simulink model "egnition_New_updated_shiva"  (R2019b)
settings: Solver=ode1  StartTime=0.0  StopTime=170  FixedStep=0.01  RelTol=1e-3
undefined symbols (not defined in the file or in its folder): BezierCurves, BezierLength, Constants, Driver, Ln, magnitude, v31
libraries: simulink_extras x3, simulink x2
(part 1 of 2)
settings Model: Creator=sivanand.shankar  LastModifiedBy=pradh
settings SolverCC: AlgebraicLoopSolver=LineSearch
settings DataIOCC: ReturnWorkspaceOutputs=off
settings DebuggingCC: ArithmeticOperatorsInVariantConditions=warning
settings SFSimCC: CustomCodeUndefinedFunction=UseInterfaceOnly

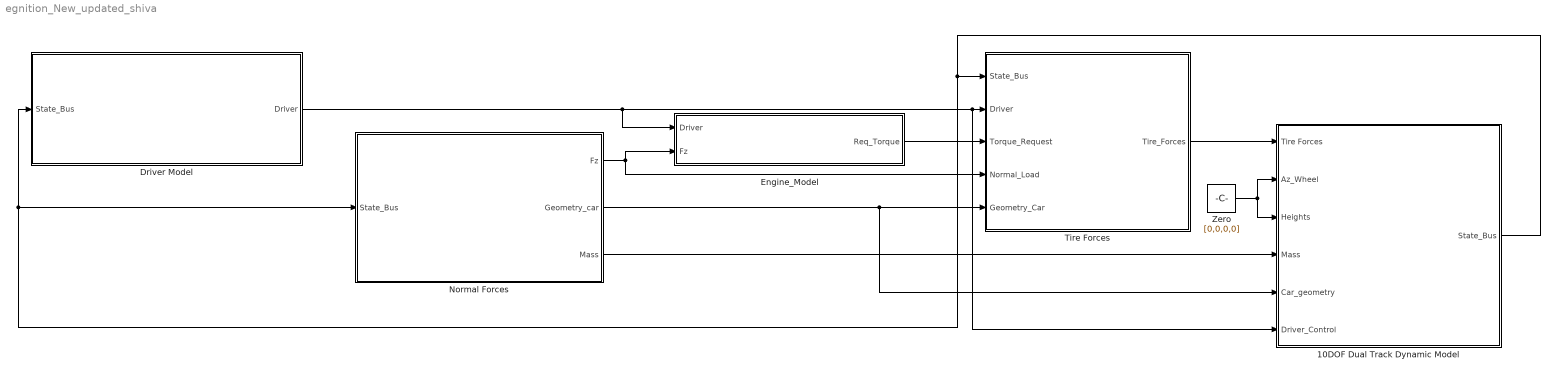
== system egnition_New_updated_shiva ==
  10DOF Dual Track Dynamic Model : Subsystem
  Driver Model : Subsystem
  Engine_Model : Subsystem
  Normal Forces : Subsystem
  "Tire Forces " : Subsystem
  Zero : Constant  Value=[0,0,0,0]
  wires:
  Normal Forces/1(Fz) -> "Tire Forces "/4(Normal_Load), Engine_Model/2(Fz)
  Normal Forces/2(Geometry_car) -> 10DOF Dual Track Dynamic Model/5(Car_geometry), "Tire Forces "/5(Geometry_Car)
  Driver Model/1(Driver) -> Engine_Model/1("Driver "), 10DOF Dual Track Dynamic Model/6(Driver_Control), "Tire Forces "/2(Driver)
  Engine_Model/1(Req_Torque) -> "Tire Forces "/3(Torque_Request)
  "Tire Forces "/1(Tire_Forces) -> 10DOF Dual Track Dynamic Model/1(Tire Forces)
  10DOF Dual Track Dynamic Model/1(State_Bus) -> Driver Model/1(State_Bus), Normal Forces/1(State_Bus), "Tire Forces "/1(State_Bus)
  Zero/1 -> 10DOF Dual Track Dynamic Model/3(Heights), 10DOF Dual Track Dynamic Model/2(Az_Wheel)
  Normal Forces/3(Mass) -> 10DOF Dual Track Dynamic Model/4(Mass)

== system egnition_New_updated_shiva/10DOF Dual Track Dynamic Model ==
  Tire Forces : Inport
  Az_Wheel : Inport  Port=2
  Heights : Inport  Port=3
  Mass : Inport  Port=4
  Car_geometry : Inport  Port=5
  Driver_Control : Inport  Port=6
  Bus Selector : BusSelector  OutputSignals=Fx,Fy
  Vehicle Model : Subsystem
  State_Bus : Outport  VectorParamsAs1DForOutWhenUnconnected=off
  wires:
  Bus Selector/2 -> Vehicle Model/2(Fy)  "<Fy>"
  Bus Selector/1 -> Vehicle Model/1(Fx)  "<Fx>"
  Tire Forces/1 -> Bus Selector/1
  Driver_Control/1 -> Vehicle Model/3(Wheel Angle)
  Heights/1 -> Vehicle Model/7(Heights)
  Mass/1 -> Vehicle Model/6(Mass)
  Az_Wheel/1 -> Vehicle Model/4(Az_Wheel)
  Car_geometry/1 -> Vehicle Model/5(Car_geometry)
  Vehicle Model/1(States Of the Car) -> State_Bus/1

== system egnition_New_updated_shiva/Driver Model ==
  State_Bus : Inport
  Bus Creator : BusCreator  Inputs=3
  Bus Selector : BusSelector  OutputSignals=Velocity.Vx
  Longitudinal Controller : Subsystem  VariantControl=Manual_Driving
  lateral Controller : Subsystem
  Driver : Outport  VectorParamsAs1DForOutWhenUnconnected=off
  wires:
  Longitudinal Controller/2(Brake (0-1)) -> Bus Creator/2  "BrakePos"
  Longitudinal Controller/1(Throttle (0-1)) -> Bus Creator/1  "ThrottlePos"
  State_Bus/1 -> lateral Controller/1("Input Bus "), Bus Selector/1
  Bus Creator/1 -> Driver/1
  Bus Selector/1 -> Longitudinal Controller/1(Drive Velocity)  "<Vx>"
  lateral Controller/1(Steering_Angle) -> Bus Creator/3  "WheelAngle"
  lateral Controller/2(Output) -> Longitudinal Controller/2(length)

== system egnition_New_updated_shiva/Engine_Model ==
  "Driver " : Inport
  Fz : Inport  Port=2
  Add : Sum  Inputs=4
  Bus Creator : BusCreator  Inputs=4
  Bus Selector : BusSelector  OutputSignals=Fz_total.FZ_FL,Fz_total.FZ_FR,Fz_total.FZ_RL,Fz_total.FZ_RR
  Bus Selector1 : BusSelector  OutputSignals=ThrottlePos,BrakePos
  Divide{,1..3} (4 alike) : Product  Inputs=*/
  MATLAB Function : MATLAB Function  TreatAsAtomicUnit=on
  Max Torque for the Car(Nm) : Constant  Value=Constants.driving_param.front_peak_torque*4
  Product{,1..3} (4 alike) : Product
  Saturation{,1..3} (4 alike) : Saturate  UpperLimit=Constants.driving_param.front_peak_torque  LowerLimit=-Constants.driving_param.front_peak_torque
  Scope : Scope  NumInputPorts=4
  Req_Torque : Outport  VectorParamsAs1DForOutWhenUnconnected=off
  wires:
  Saturation1/1 -> Scope/2, Bus Creator/2  "Vectored Torque FR"
  Bus Creator/1 -> Req_Torque/1
  Product1/1 -> Saturation1/1
  Bus Selector/1 -> Divide/1, Add/1  "<FZ_FL>"
  Product2/1 -> Saturation2/1
  Saturation/1 -> Scope/1, Bus Creator/1  "Vectored Torque FL"
  Product3/1 -> Saturation3/1
  Saturation3/1 -> Scope/4, Bus Creator/4  "Vectored Torque RR"
  Product/1 -> Saturation/1
  Divide2/1 -> Product2/1
  Saturation2/1 -> Scope/3, Bus Creator/3  "Vectored Torque RL"
  Bus Selector/2 -> Divide1/1, Add/2  "<FZ_FR>"
  Divide/1 -> Product/1
  Add/1 -> Divide1/2, Divide/2, Divide2/2, Divide3/2
  Bus Selector/4 -> Divide3/1, Add/4  "<FZ_RR>"
  Divide3/1 -> Product3/1
  Divide1/1 -> Product1/1
  Bus Selector/3 -> Divide2/1, Add/3  "<FZ_RL>"
  Fz/1 -> Bus Selector/1
  Max Torque for the Car(Nm)/1 -> MATLAB Function/3(T_peak)
  Bus Selector1/1 -> MATLAB Function/1(TP)  "<ThrottlePos>"
  Bus Selector1/2 -> MATLAB Function/2(BP)  "<BrakePos>"
  "Driver "/1 -> Bus Selector1/1
  MATLAB Function/1(Requested_Torque) -> Product/2, Product1/2, Product3/2, Product2/2

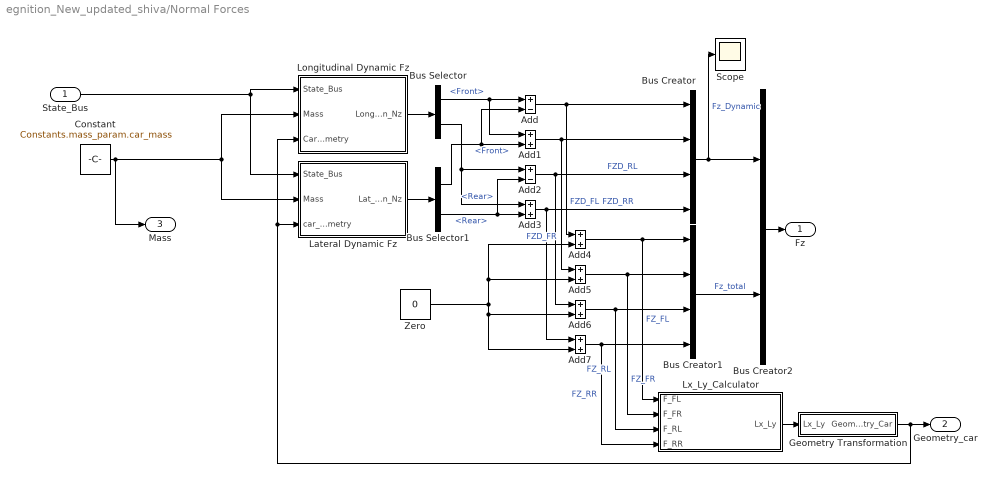
== system egnition_New_updated_shiva/Normal Forces ==
  State_Bus : Inport
  Add : Sum  Inputs=+-
  Add{1,3..7} (6 alike) : Sum
  Add2 : Sum  Inputs=+-
  Bus Creator : BusCreator  Inputs=4
  Bus Creator1 : BusCreator  Inputs=4
  Bus Creator2 : BusCreator  Inputs=2
  Bus Selector : BusSelector  OutputSignals=Front,Rear
  Bus Selector1 : BusSelector  OutputSignals=Front,Rear
  Constant : Constant  Value=Constants.mass_param.car_mass
  Geometry Transformation : Subsystem
  Lateral Dynamic Fz : Subsystem  mask{a_s=Constants.dim_param_mass.distance_of_sprung_cg_from_rear_axle, W_s=Constants.mass_param.sprung_mass, K_F=Constants.roll_param.front_roll_stiffness, L_cgr=Constants.dim_param_mass.distance_sprung_mass_cg_and_roll_axis, K_R=Constants.roll_param.rear_roll_stiffness, H_s=Constants.dim_param_mass.height_front_unsprung_cg, Z_RF=Constants.roll_param.front_roll_center_height, Z_RR=Constants.roll_param.rear_roll_center_height, W_uF=Constants.mass_param.front_unsprung_mass, W_uR=Constants.mass_param.rear_unsprung_mass, Z_uF=Constants.dim_param_mass.height_front_unsprung_cg, Z_uR=Constants.dim_param_mass.height_rear_unsprung_cg}
      mask prompts: a_s "Distance of sprung cg from rear axle"; W_s "Sprung Mass"; K_F "Front Roll Stiffness"; L_cgr "Distance from Sprung mass CG to Roll Axis"; K_R "Rear Roll Stiffness"; H_s "Unsprung Mass CG Height"; Z_RF "Roll Centric Height Front"; Z_RR "Roll Centric Height Rear"; W_uF "Front UnSprung Mass"; W_uR "Rear UnSprung Mass"; Z_uF "Front Unsprung CG Height"; Z_uR "Rear Unsprung CG Height"
  Longitudinal Dynamic Fz : Subsystem  mask{CG_Height=Constants.dim_param.cg_height}
      mask prompts: CG_Height "Height CoG"
  Lx_Ly_Calculator : Subsystem  mask{wb=Constants.dim_param.wheel_base, wt_FA=Constants.dim_param.front_track, wt_RA=Constants.dim_param.rear_track}
      mask prompts: wb "Wheel base [m]"; wt_FA "Wheel track [m] - front axle"; wt_RA "Wheel track [m] - rear axle"
      mask DialogControl DescGroupVar Prompt: Corner position calculation
      mask DialogControl DescTextVar Prompt: Calculates the height of the vehicle corners based on the height, the roll angle and the pitch at the center of gravity
  Scope : Scope
  Zero : Constant  Value=0  OutDataTypeStr=Inherit: Inherit via back propagation
  Fz : Outport  VectorParamsAs1DForOutWhenUnconnected=off
  Geometry_car : Outport  Port=2  VectorParamsAs1DForOutWhenUnconnected=off
  Mass : Outport  Port=3  VectorParamsAs1DForOutWhenUnconnected=off
  wires:
  Geometry Transformation/1(Geometry_Car) -> Geometry_car/1, Lateral Dynamic Fz/3(car_Geometry), Longitudinal Dynamic Fz/3(Car_Geometry)
  Lx_Ly_Calculator/1(Lx_Ly) -> Geometry Transformation/1(Lx_Ly)
  Bus Creator2/1 -> Fz/1
  Bus Creator/1 -> Scope/1, Bus Creator2/1  "Fz_Dynamic"
  Bus Selector1/1 -> Add1/2, Add/2  "<Front>"
  Bus Selector1/2 -> Add3/2, Add2/2  "<Rear>"
  Add1/1 -> Bus Creator/2, Add5/1  "FZD_FR"
  Add2/1 -> Bus Creator/3, Add6/1  "FZD_RL"
  Add3/1 -> Bus Creator/4, Add7/1  "FZD_RR"
  Bus Selector/2 -> Add3/1, Add2/1  "<Rear>"
  Bus Selector/1 -> Add/1, Add1/1  "<Front>"
  Lateral Dynamic Fz/1(Lat_Dyn_Nz) -> Bus Selector1/1
  Longitudinal Dynamic Fz/1(Long_Dyn_Nz) -> Bus Selector/1
  State_Bus/1 -> Lateral Dynamic Fz/1(State_Bus), Longitudinal Dynamic Fz/1(State_Bus)
  Add4/1 -> Bus Creator1/1, Lx_Ly_Calculator/1(F_FL)  "FZ_FL"
  Add5/1 -> Bus Creator1/2, Lx_Ly_Calculator/2(F_FR)  "FZ_FR"
  Add6/1 -> Bus Creator1/3, Lx_Ly_Calculator/3(F_RL)  "FZ_RL"
  Add7/1 -> Bus Creator1/4, Lx_Ly_Calculator/4(F_RR)  "FZ_RR"
  Add/1 -> Add4/1, Bus Creator/1  "FZD_FL"
  Bus Creator1/1 -> Bus Creator2/2  "Fz_total"
  Constant/1 -> Mass/1, Lateral Dynamic Fz/2(Mass), Longitudinal Dynamic Fz/2(Mass)
  Zero/1 -> Add7/2, Add6/2, Add5/2, Add4/2

== system egnition_New_updated_shiva/Tire Forces  ==
  State_Bus : Inport
  Driver : Inport  Port=2
  Torque_Request : Inport  Port=3
  Normal_Load : Inport  Port=4
  Geometry_Car : Inport  Port=5
  Bus Creator : BusCreator  Inputs=2
  Tire Model : Subsystem  mask{Radius=Constants.wheel_param.wheel_radius}
      mask prompts: Radius "Radius of the wheel"
  Tire_Forces : Outport  VectorParamsAs1DForOutWhenUnconnected=off
  wires:
  Tire Model/1(Fx) -> Bus Creator/1  "Fx"
  Bus Creator/1 -> Tire_Forces/1
  Tire Model/2(Fy) -> Bus Creator/2  "Fy"
  Normal_Load/1 -> Tire Model/5(Nz)
  Torque_Request/1 -> Tire Model/4(Req Torrque)
  Driver/1 -> Tire Model/3(Driver)
  Geometry_Car/1 -> Tire Model/2(Geometry_Car)
  State_Bus/1 -> Tire Model/1(State Bus)

== system egnition_New_updated_shiva/10DOF Dual Track Dynamic Model/Vehicle Model ==
  Fx : Inport
  Fy : Inport  Port=2
  Wheel Angle : Inport  Port=3
  Az_Wheel : Inport  Port=4
  Car_geometry : Inport  Port=5
  Mass : Inport  Port=6
  Heights : Inport  Port=7
  Bus Creator : BusCreator  Inputs=2
  Bus Creator1 : BusCreator  Inputs=3
  Bus Creator2 : BusCreator  Inputs=3
  Bus Creator3 : BusCreator  Inputs=3
  Bus Creator4 : BusCreator  Inputs=4
  Bus Creator5 : BusCreator  Inputs=2
  Bus Selector : BusSelector  OutputSignals=WheelAngle
  "Roll And Pitch " : Subsystem  mask{Ts=25}
      mask prompts: Ts "Sampling Time of the car sensors"
  Vehicle Model : Subsystem  mask{Jz=Constants.other_param.Moment_of_Inertia, Radius=Constants.wheel_param.wheel_radius}
      mask prompts: Jz "Moment of Inertia around Z axis"; Radius "Radius of the tire"
      mask TypeOptions Jz: Moment_of_Inertia_Z/Value
  States Of the Car : Outport  VectorParamsAs1DForOutWhenUnconnected=off
  wires:
  Az_Wheel/1 -> Vehicle Model/6(Az)
  Mass/1 -> Vehicle Model/5(Mass)
  Car_geometry/1 -> Vehicle Model/4(Car_Geometry)
  Fy/1 -> Vehicle Model/2("Fy ")
  Fx/1 -> Vehicle Model/1(Fx)
  Vehicle Model/4(Velocity_Y) -> Bus Creator1/2  "Vy"
  Vehicle Model/3(Velocity_X) -> Bus Creator1/1  "Vx"
  Vehicle Model/5(Yaw Rate) -> Bus Creator1/3  "Psi_Dot"
  Vehicle Model/1(Acceleration_X) -> Bus Creator/1  "Ax"
  Bus Creator/1 -> Bus Creator4/1  "Acceleration"
  Bus Creator1/1 -> Bus Creator4/2  "Velocity"
  Bus Creator2/1 -> Bus Creator4/3  "Position"
  Bus Creator4/1 -> States Of the Car/1
  Wheel Angle/1 -> Bus Selector/1
  Bus Selector/1 -> Vehicle Model/3(Wheel_Angle)  "<WheelAngle>"
  Vehicle Model/7(Position_Y) -> Bus Creator2/2  "Y"
  Vehicle Model/6(Position_X) -> Bus Creator2/1  "X"
  Vehicle Model/8(Position_Z) -> Bus Creator2/3  "Z"
  Vehicle Model/9(Yaw Angle) -> Bus Creator3/1  "Psi"
  Heights/1 -> "Roll And Pitch "/1(Heights)
  Vehicle Model/2(Acceleration_Y) -> Bus Creator/2  "Ay"
  Bus Creator3/1 -> Bus Creator4/4  "Angle"
  Bus Creator5/1 -> Vehicle Model/7(Roll and Pitch)  "Angle"
  "Roll And Pitch "/1(Pitch) -> Bus Creator5/1, Bus Creator3/2  "Theta"
  "Roll And Pitch "/2(Roll) -> Bus Creator5/2, Bus Creator3/3  "Phi"

== system egnition_New_updated_shiva/Driver Model/Longitudinal Controller ==
  note: Velocity Input
  Drive Velocity : Inport
  length : Inport  Port=2
  1-D Lookup Table : Lookup_n-D  NumberOfTableDimensions=1  BreakpointsForDimension1=Ln  Table=v31  InternalRulePriority=Speed  RndMeth=Simplest  InputSameDT=on
  B % to Decimal : Gain  Gain=-0.01
  Brake extractor : Saturate  UpperLimit=0  LowerLimit=-100
  Constant1 : Constant  Value=1.53
  Initialization : Step  Time=Constants.initial_param.initialization_velocity  After=Constants.initial_param.step_val
  Longitudinal PID : simulink/Continuous/PID Controller  Controller=PI  Form=Parallel  TimeDomain=Continuous-time  SampleTime=-1  IntegratorMethod=Forward Euler  FilterMethod=Forward Euler  ControllerParametersSource=internal  P=50  I=2  D=Driver.Long.PID.Kd  UseFilter=on  N=Driver.Long.PID.N  TunerSelectOption=Transfer Function Based (PID Tuner App)  InitialConditionSource=internal  InitialConditionForIntegrator=0  InitialConditionForFilter=0  DifferentiatorICPrevScaledInput=0  ExternalReset=none  TrackingMode=off  Kt=1  LimitOutput=off  UpperSaturationLimit=inf  LowerSaturationLimit=-inf  LinearizeAsGain=on  AntiWindupMode=none  Kb=1  POutMin=[]  POutMax=[]  IOutMin=[]  IOutMax=[]  DOutMin=[]  DOutMax=[]  NOutMin=[]  NOutMax=[]  SumOutMin=[]  SumOutMax=[]  SaturationOutMin=[]  SaturationOutMax=[]  PParamMin=[]  PParamMax=[]  IParamMin=[]  IParamMax=[]  DParamMin=[]  DParamMax=[]  NParamMin=[]  NParamMax=[]  KbParamMin=[]  KbParamMax=[]  KtParamMin=[]  KtParamMax=[]  KbOutMin=[]  KbOutMax=[]  KtOutMin=[]  KtOutMax=[]  IntegratorOutMin=[]  IntegratorOutMax=[]  FilterOutMin=[]  FilterOutMax=[]  SumI1OutMin=[]  SumI1OutMax=[]  SumI2OutMin=[]  SumI2OutMax=[]  SumI3OutMin=[]  SumI3OutMax=[]  SumI4OutMin=[]  SumI4OutMax=[]  SumDOutMin=[]  SumDOutMax=[]  DifferentiatorOutMin=[]  DifferentiatorOutMax=[]  FilterDiffOutCoefMin=[]  FilterDiffOutCoefMax=[]  ReciprocalOutMin=[]  ReciprocalOutMax=[]  SumDenOutMin=[]  SumDenOutMax=[]  SumNumOutMin=[]  SumNumOutMax=[]  DivideOutMin=[]  DivideOutMax=[]  IntegratorContinuousStateAttributes=''  IntegratorStateMustResolveToSignalObject=off  IntegratorRTWStateStorageClass=Auto  FilterContinuousStateAttributes=''  FilterStateMustResolveToSignalObject=off  FilterRTWStateStorageClass=Auto  ParallelPVariant=InternalParameters  IdealPVariant=Disabled  IVariant=InternalParameters  DVariant=Disabled  IntegratorVariant=Continuous  SatVariant=Disabled  AWVariant=Passthrough  PCopyVariant=Disabled  TRVariant=Disabled  FdbkBlocksVariant=Forward  IdealPFdbkVariant=Disabled  SatFdbkVariant=Disabled  DerivativeFilterVariant=Disabled  NVariant=Disabled  NCopyVariant=Disabled_SignalSpec  FilterICVariant=Disabled  IntegratorICVariant=InternalICs  ExternalResetVariant=Disabled  TRSumVariant=Passthrough  SumFdbkVariant=Disabled  SumVariant=Sum_PI
  Manual Input : Constant  Value=35
  Manual Switch : ManualSwitch  CurrentSetting=0
  Max_Velocity Saturation : Saturate  UpperLimit=50  LowerLimit=0
  Product : Product
  Scope1 : Scope
  Scope2 : Scope
  Sum : Sum  Inputs=-+
  Sum1 : Sum  Inputs=|++
  T % to Decimal : Gain  Gain=0.01
  Throttle extractor : Saturate  UpperLimit=100  LowerLimit=0
  kmph to mps : Gain  Gain=1/3.6
  kmph to mps2 : Gain  Gain=3.6
  Throttle (0-1) : Outport  VectorParamsAs1DForOutWhenUnconnected=off
  Brake (0-1) : Outport  Port=2  VectorParamsAs1DForOutWhenUnconnected=off
  wires:
  Product/1 -> Max_Velocity Saturation/1, Scope1/1
  Throttle extractor/1 -> T % to Decimal/1
  Longitudinal PID/1 -> Brake extractor/1, Throttle extractor/1
  Brake extractor/1 -> B % to Decimal/1
  kmph to mps/1 -> Product/1  "Reference Speed"
  Manual Switch/1 -> kmph to mps/1
  Manual Input/1 -> Manual Switch/2
  Initialization/1 -> Product/2
  B % to Decimal/1 -> Brake (0-1)/1
  Max_Velocity Saturation/1 -> Sum/2
  Sum/1 -> Longitudinal PID/1
  Drive Velocity/1 -> Sum/1  "Actual_Speed"
  T % to Decimal/1 -> Scope2/1, Throttle (0-1)/1
  1-D Lookup Table/1 -> kmph to mps2/1  "Reference Speed"
  Sum1/1 -> 1-D Lookup Table/1
  Constant1/1 -> Sum1/2
  length/1 -> Sum1/1
  kmph to mps2/1 -> Manual Switch/1  "Reference Speed"

== system egnition_New_updated_shiva/Driver Model/lateral Controller ==
  "Input Bus " : Inport
  BezierPathReference : MATLAB Function  TreatAsAtomicUnit=on
  Bus Selector : BusSelector  OutputSignals=Angle.Psi
  Bus Selector1 : BusSelector  OutputSignals=Position.X,Position.Y,Position.Z
  Bus Selector2 : BusSelector  OutputSignals=Velocity.Psi_Dot
  Bus Selector3 : BusSelector  OutputSignals=Velocity.Vx
  Bus Selector4 : BusSelector  OutputSignals=Angle.Psi
  Constant : Constant  Value=0.001
  Constant1 : Constant  Value=BezierCurves
  Constant2 : Constant  Value=BezierLength
  IC{,1..2,4} (4 alike) : InitialCondition  Value=0
  IC3 : InitialCondition  Value=[0;0;0]
  Mux : Mux  Inputs=3
  Scope2 : Scope  NumInputPorts=3
  Subsystem : Subsystem
  Steering_Angle : Outport  VectorParamsAs1DForOutWhenUnconnected=off
  Output : Outport  Port=2
  wires:
  BezierPathReference/1(ey) -> IC/1, Scope2/1  "ey"
  Constant1/1 -> BezierPathReference/4(bezierCurves)
  IC3/1 -> BezierPathReference/1(pCar)
  "Input Bus "/1 -> Bus Selector3/1, Bus Selector4/1, Bus Selector2/1, Bus Selector1/1, Bus Selector/1
  Mux/1 -> IC3/1
  IC1/1 -> Subsystem/2(e_gamma)
  IC2/1 -> BezierPathReference/2(yawCar)
  Bus Selector1/3 -> Mux/3  "<Z>"
  Bus Selector/1 -> IC2/1  "<Psi>"
  BezierPathReference/2(eYaw) -> IC1/1, Scope2/2  "eyaw"
  IC/1 -> Subsystem/1(ey)
  Constant2/1 -> BezierPathReference/5(bezierLength)
  Bus Selector1/1 -> Mux/1  "<X>"
  Constant/1 -> BezierPathReference/3(tol)
  Bus Selector1/2 -> Mux/2  "<Y>"
  BezierPathReference/3(kappa) -> IC4/1, Scope2/3
  IC4/1 -> Subsystem/3(kappa)
  Bus Selector2/1 -> Subsystem/4(psi_dot)  "<Psi_Dot>"
  Bus Selector3/1 -> Subsystem/5(dx_C_dt)  "<Vx>"
  Bus Selector4/1 -> Subsystem/6(psi)  "<Psi>"
  Subsystem/1(delta_fb) -> Steering_Angle/1
  BezierPathReference/4(lengh) -> Output/1  "length"

== system egnition_New_updated_shiva/Normal Forces/Geometry Transformation ==
  Lx_Ly : Inport
  Bus Creator : BusCreator  Inputs=5
  Constant : Constant  Value=Constants.dim_param.dist_cg_front
  Constant1 : Constant  Value=Constants.dim_param.dist_cg_rear
  Constant2 : Constant  Value=Constants.dim_param.front_track
  Constant3 : Constant  Value=Constants.dim_param.rear_track
  Constant4 : Constant  Value=Constants.dim_param.wheel_base
  Terminator : Terminator
  Geometry_Car : Outport  VectorParamsAs1DForOutWhenUnconnected=off
  wires:
  Bus Creator/1 -> Geometry_Car/1
  Constant/1 -> Bus Creator/1  "Lf"
  Constant1/1 -> Bus Creator/2  "Lr"
  Constant2/1 -> Bus Creator/3  "Tf"
  Constant3/1 -> Bus Creator/4  "Tr"
  Constant4/1 -> Bus Creator/5  "Wb"
  Lx_Ly/1 -> Terminator/1

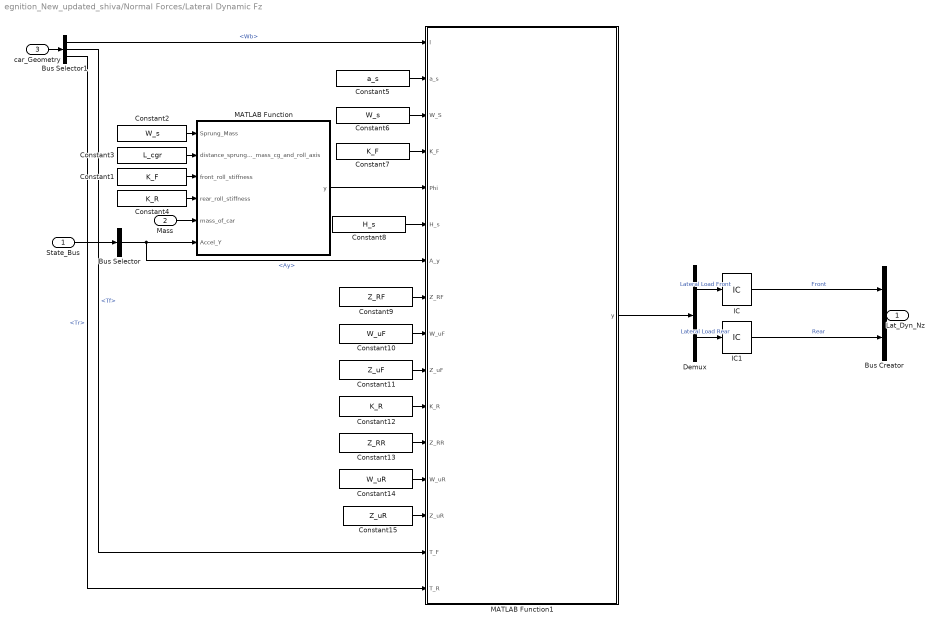
== system egnition_New_updated_shiva/Normal Forces/Lateral Dynamic Fz ==
  State_Bus : Inport
  Mass : Inport  Port=2
  car_Geometry : Inport  Port=3
  Bus Creator : BusCreator  Inputs=2
  Bus Selector : BusSelector  OutputSignals=Acceleration.Ay
  Bus Selector1 : BusSelector  OutputSignals=Wb,Tf,Tr
  Constant1 : Constant  Value=K_F
  Constant10 : Constant  Value=W_uF  VectorParams1D=off
  Constant11 : Constant  Value=Z_uF  VectorParams1D=off
  Constant12 : Constant  Value=K_R  VectorParams1D=off
  Constant13 : Constant  Value=Z_RR  VectorParams1D=off
  Constant14 : Constant  Value=W_uR  VectorParams1D=off
  Constant15 : Constant  Value=Z_uR  VectorParams1D=off
  Constant2 : Constant  Value=W_s
  Constant3 : Constant  Value=L_cgr
  Constant4 : Constant  Value=K_R
  Constant5 : Constant  Value=a_s
  Constant6 : Constant  Value=W_s  VectorParams1D=off
  Constant7 : Constant  Value=K_F  VectorParams1D=off
  Constant8 : Constant  Value=H_s  VectorParams1D=off
  Constant9 : Constant  Value=Z_RF  VectorParams1D=off
  Demux : Demux  Outputs=2
  IC : InitialCondition  Value=0
  IC1 : InitialCondition  Value=0
  MATLAB Function : MATLAB Function  TreatAsAtomicUnit=on
  MATLAB Function1 : MATLAB Function  TreatAsAtomicUnit=on
  Lat_Dyn_Nz : Outport  VectorParamsAs1DForOutWhenUnconnected=off
  wires:
  Demux/2 -> IC1/1  "Lateral Load Rear"
  Constant13/1 -> MATLAB Function1/12(Z_RR)
  Constant6/1 -> MATLAB Function1/3(W_S)
  MATLAB Function1/1(y) -> Demux/1
  Constant12/1 -> MATLAB Function1/11(K_R)
  IC1/1 -> Bus Creator/2  "Rear"
  Bus Creator/1 -> Lat_Dyn_Nz/1
  Constant7/1 -> MATLAB Function1/4(K_F)
  Demux/1 -> IC/1  "Lateral Load Front"
  IC/1 -> Bus Creator/1  "Front"
  Bus Selector1/3 -> MATLAB Function1/16(T_R)  "<Tr>"
  Constant8/1 -> MATLAB Function1/6(H_s)
  Constant10/1 -> MATLAB Function1/9(W_uF)
  Constant3/1 -> MATLAB Function/2(distance_sprung_mass_cg_and_roll_axis)
  Bus Selector1/1 -> MATLAB Function1/1(l)  "<Wb>"
  Constant1/1 -> MATLAB Function/3(front_roll_stiffness)
  Constant14/1 -> MATLAB Function1/13(W_uR)
  MATLAB Function/1(y) -> MATLAB Function1/5(Phi)
  Constant11/1 -> MATLAB Function1/10(Z_uF)
  Constant15/1 -> MATLAB Function1/14(Z_uR)
  Constant2/1 -> MATLAB Function/1(Sprung_Mass)
  Bus Selector/1 -> MATLAB Function1/7(A_y), MATLAB Function/6(Accel_Y)  "<Ay>"
  Bus Selector1/2 -> MATLAB Function1/15(T_F)  "<Tf>"
  Constant4/1 -> MATLAB Function/4(rear_roll_stiffness)
  Constant9/1 -> MATLAB Function1/8(Z_RF)
  Mass/1 -> MATLAB Function/5(mass_of_car)
  State_Bus/1 -> Bus Selector/1
  car_Geometry/1 -> Bus Selector1/1
  Constant5/1 -> MATLAB Function1/2(a_s)

== system egnition_New_updated_shiva/Normal Forces/Longitudinal Dynamic Fz ==
  State_Bus : Inport
  Mass : Inport  Port=2
  Car_Geometry : Inport  Port=3
  Bus Creator : BusCreator  Inputs=2
  Bus Selector : BusSelector  OutputSignals=Velocity.Vx,Acceleration.Ax
  Bus Selector1 : BusSelector  OutputSignals=Lr,Lf,Wb
  Constant5 : Constant  Value=CG_Height
  Demux : Demux  Outputs=2
  IC : InitialCondition  Value=Constants.dim_param.wheel_base
  IC1 : InitialCondition  Value=Constants.mass_param.car_mass*9.81/4
  IC2 : InitialCondition  Value=Constants.mass_param.car_mass*9.81/4
  MATLAB Function : MATLAB Function  TreatAsAtomicUnit=on
  Saturation : Saturate  UpperLimit=1600  LowerLimit=-1600
  Long_Dyn_Nz : Outport  VectorParamsAs1DForOutWhenUnconnected=off
  wires:
  Bus Selector/1 -> MATLAB Function/1(V_COG)  "<Vx>"
  MATLAB Function/1(y) -> Saturation/1
  IC1/1 -> Bus Creator/1  "Front"
  Demux/1 -> IC1/1  "Longitudinal Load FL"
  Bus Creator/1 -> Long_Dyn_Nz/1
  Bus Selector1/3 -> IC/1  "<Wb>"
  Bus Selector/2 -> MATLAB Function/2(Accel_X)  "<Ax>"
  Car_Geometry/1 -> Bus Selector1/1
  Constant5/1 -> MATLAB Function/6(H_COG)
  Mass/1 -> MATLAB Function/3(W)
  State_Bus/1 -> Bus Selector/1
  Demux/2 -> IC2/1  "Longitudinal Lod FR"
  IC/1 -> MATLAB Function/7(Wb)
  Bus Selector1/1 -> MATLAB Function/4(C)  "<Lr>"
  Bus Selector1/2 -> MATLAB Function/5(B)  "<Lf>"
  IC2/1 -> Bus Creator/2  "Rear"
  Saturation/1 -> Demux/1

== system egnition_New_updated_shiva/Normal Forces/Lx_Ly_Calculator ==
  F_FL : Inport
  F_FR : Inport  Port=2
  F_RL : Inport  Port=3
  F_RR : Inport  Port=4
  Constant : Constant  Value=wb
  Constant1 : Constant  Value=wt_FA
  Constant2 : Constant  Value=wt_RA
  MATLAB Function : MATLAB Function  TreatAsAtomicUnit=on
  Lx_Ly : Outport  VectorParamsAs1DForOutWhenUnconnected=off
  wires:
  Constant2/1 -> MATLAB Function/7(Rear_track)
  Constant1/1 -> MATLAB Function/6(Front_track)
  Constant/1 -> MATLAB Function/5(Wheel_Base)
  F_RR/1 -> MATLAB Function/4(W_RR)
  F_RL/1 -> MATLAB Function/3(W_RL)
  F_FL/1 -> MATLAB Function/1(W_FL)
  MATLAB Function/1(y) -> Lx_Ly/1
  F_FR/1 -> MATLAB Function/2(W_FR)

== system egnition_New_updated_shiva/Tire Forces /Tire Model ==
  State Bus : Inport
  Geometry_Car : Inport  Port=2
  Driver : Inport  Port=3
  Req Torrque : Inport  Port=4
  Nz : Inport  Port=5
  " Longitudinal  Force" : Subsystem
  Bus Selector : BusSelector  OutputSignals=WheelAngle
  Lateral Forces : Subsystem
  Side Slip angle calculation : Subsystem
  Slip angle calculation : Subsystem
  Wheel Model1 : Subsystem  mask{Iyy=(0.5)*7*(Constants.wheel_param.wheel_radius)*(Constants.wheel_param.wheel_radius)}
      mask prompts: Iyy "Intertia around Y axis"
  "Wheel slip calculation " : Subsystem
  co efficient of friction calculation : Subsystem
  "wheel velocities " : Subsystem  mask{Radius=Constants.wheel_param.wheel_radius}
      mask prompts: Radius "Radius of the wheel"
  Fx : Outport  VectorParamsAs1DForOutWhenUnconnected=off
  Fy : Outport  Port=2  VectorParamsAs1DForOutWhenUnconnected=off
  wires:
  Bus Selector/1 -> Lateral Forces/1(Steering Angle), " Longitudinal  Force"/2(Steering Angle)  "<WheelAngle>"
  Geometry_Car/1 -> Slip angle calculation/2(Geometry_car), "wheel velocities "/4(Car_Geometry)
  "wheel velocities "/1(Wheel Velocity X) -> Wheel Model1/4(Vx), "Wheel slip calculation "/3(Wheel Velocity X)
  " Longitudinal  Force"/1(Fx) -> Wheel Model1/2(Fx)
  Lateral Forces/1(Fy) -> Fy/1
  co efficient of friction calculation/1(Mew) -> Lateral Forces/3(Mew)
  State Bus/1 -> Slip angle calculation/3(Input Bus), Wheel Model1/1(State_Bus), "wheel velocities "/2(Input Bus), Side Slip angle calculation/1(Input Bus)
  Nz/1 -> Wheel Model1/5(Fz), co efficient of friction calculation/2(Fz), Lateral Forces/4(FZ)
  Side Slip angle calculation/1(Side Slip Angle) -> Slip angle calculation/4(Side slip angle), "wheel velocities "/1("Side slip ")
  "Wheel slip calculation "/1(" Slip") -> co efficient of friction calculation/1("Resultant Slip ")
  Wheel Model1/2(Long_Driving_Torque) -> Fx/1
  Lateral Forces/2(Fws) -> " Longitudinal  Force"/1(Fws)
  Wheel Model1/1(V_Omega) -> "wheel velocities "/3(Wheel_Omega)
  Slip angle calculation/1(Slip Angle) -> Lateral Forces/2(Slip Angle), "Wheel slip calculation "/2("Slip Angle "), " Longitudinal  Force"/4(Slip Angle)
  Driver/1 -> Bus Selector/1, "Wheel slip calculation "/1(Driver), Slip angle calculation/1("Driver ")
  Req Torrque/1 -> Wheel Model1/3(Req_Torque)
  Lateral Forces/3(Fwl) -> " Longitudinal  Force"/3("Fwl ")

== system egnition_New_updated_shiva/10DOF Dual Track Dynamic Model/Vehicle Model/Roll And Pitch  ==
  Heights : Inport
  Add1 : Sum
  Add2 : Sum
  Add3 : Sum  Inputs=+-
  Add5 : Sum  Inputs=+-
  Atan : Trigonometry  Operator=atan
  Atan1 : Trigonometry  Operator=atan
  Atan2 : Trigonometry  Operator=atan
  Demux : Demux
  Gain : Gain  Gain=1/Constants.dim_param.wheel_base
  Gain1 : Gain  Gain=1/Constants.dim_param.front_track
  Gain2 : Gain  Gain=0.5
  Gain3 : Gain  Gain=0.5
  Gain4 : Gain  Gain=1/Constants.dim_param.rear_track
  Gain5 : Gain  Gain=-0.5
  Scope : Scope  NumInputPorts=2
  Subtract : Sum  Inputs=-+
  Subtract1 : Sum
  Transfer Fcn{,1..3} (4 alike) : TransferFcn  Numerator=[Ts]  Denominator=[1 Ts]
  Pitch : Outport  VectorParamsAs1DForOutWhenUnconnected=off
  Roll : Outport  Port=2  VectorParamsAs1DForOutWhenUnconnected=off
  wires:
  Transfer Fcn3/1 -> Add2/2, Add5/2
  Transfer Fcn2/1 -> Add2/1, Add5/1
  Transfer Fcn1/1 -> Add3/2, Add1/2
  Transfer Fcn/1 -> Add1/1, Add3/1
  Atan2/1 -> Subtract1/2
  Atan1/1 -> Subtract1/1
  Gain5/1 -> Roll/1
  Gain1/1 -> Atan1/1
  Gain4/1 -> Atan2/1
  Add5/1 -> Gain4/1
  Add3/1 -> Gain1/1
  Gain/1 -> Atan/1
  Heights/1 -> Demux/1
  Demux/2 -> Transfer Fcn1/1
  Add1/1 -> Gain2/1
  Demux/4 -> Transfer Fcn3/1
  Gain3/1 -> Subtract/2
  Gain2/1 -> Subtract/1
  Demux/3 -> Transfer Fcn2/1
  Atan/1 -> Scope/1, Pitch/1
  Demux/1 -> Transfer Fcn/1
  Add2/1 -> Gain3/1
  Subtract/1 -> Gain/1
  Subtract1/1 -> Scope/2, Gain5/1

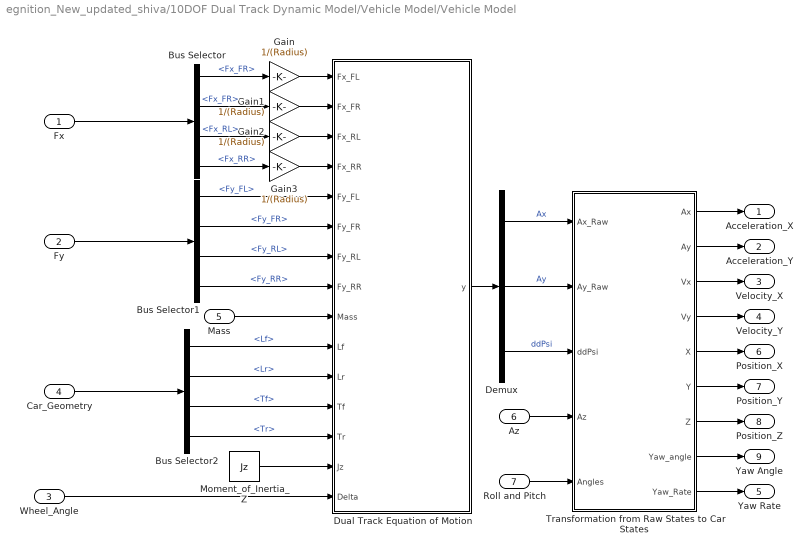
== system egnition_New_updated_shiva/10DOF Dual Track Dynamic Model/Vehicle Model/Vehicle Model ==
  Fx : Inport
  "Fy " : Inport  Port=2
  Wheel_Angle : Inport  Port=3
  Car_Geometry : Inport  Port=4
  Mass : Inport  Port=5
  Az : Inport  Port=6
  Roll and Pitch : Inport  Port=7
  Bus Selector : BusSelector  OutputSignals=Fx_FR,Fx_FR,Fx_RL,Fx_RR
  Bus Selector1 : BusSelector  OutputSignals=Fy_FL,Fy_FR,Fy_RL,Fy_RR
  Bus Selector2 : BusSelector  OutputSignals=Lf,Lr,Tf,Tr
  Demux : Demux  Outputs=3
  Dual Track Equation of Motion : MATLAB Function  TreatAsAtomicUnit=on
  Gain{,1..3} (4 alike) : Gain  Gain=1/(Radius)
  Moment_of_Inertia_Z : Constant  Value=Jz
  Transformation from Raw States to Car States : Subsystem  mask{Ts=29.5}
      mask prompts: Ts "Sampling Time of the car sensor"
  Acceleration_X : Outport  VectorParamsAs1DForOutWhenUnconnected=off
  Acceleration_Y : Outport  Port=2  VectorParamsAs1DForOutWhenUnconnected=off
  Velocity_X : Outport  Port=3  VectorParamsAs1DForOutWhenUnconnected=off
  Velocity_Y : Outport  Port=4  VectorParamsAs1DForOutWhenUnconnected=off
  Yaw Rate : Outport  Port=5  VectorParamsAs1DForOutWhenUnconnected=off
  Position_X : Outport  Port=6  VectorParamsAs1DForOutWhenUnconnected=off
  Position_Y : Outport  Port=7  VectorParamsAs1DForOutWhenUnconnected=off
  Position_Z : Outport  Port=8  VectorParamsAs1DForOutWhenUnconnected=off
  Yaw Angle : Outport  Port=9  VectorParamsAs1DForOutWhenUnconnected=off
  wires:
  Transformation from Raw States to Car States/7(Z) -> Position_Z/1
  Car_Geometry/1 -> Bus Selector2/1
  Dual Track Equation of Motion/1(y) -> Demux/1
  Bus Selector2/1 -> Dual Track Equation of Motion/10(Lf)  "<Lf>"
  Bus Selector2/2 -> Dual Track Equation of Motion/11(Lr)  "<Lr>"
  Mass/1 -> Dual Track Equation of Motion/9(Mass)
  Bus Selector2/3 -> Dual Track Equation of Motion/12(Tf)  "<Tf>"
  Bus Selector2/4 -> Dual Track Equation of Motion/13(Tr)  "<Tr>"
  Moment_of_Inertia_Z/1 -> Dual Track Equation of Motion/14(Jz)
  Fx/1 -> Bus Selector/1
  "Fy "/1 -> Bus Selector1/1
  Bus Selector1/4 -> Dual Track Equation of Motion/8(Fy_RR)  "<Fy_RR>"
  Bus Selector1/3 -> Dual Track Equation of Motion/7(Fy_RL)  "<Fy_RL>"
  Bus Selector1/2 -> Dual Track Equation of Motion/6(Fy_FR)  "<Fy_FR>"
  Bus Selector1/1 -> Dual Track Equation of Motion/5(Fy_FL)  "<Fy_FL>"
  Bus Selector/1 -> Gain/1  "<Fx_FR>"
  Bus Selector/4 -> Gain3/1  "<Fx_RR>"
  Bus Selector/3 -> Gain2/1  "<Fx_RL>"
  Bus Selector/2 -> Gain1/1  "<Fx_FR>"
  Transformation from Raw States to Car States/3(Vx) -> Velocity_X/1
  Transformation from Raw States to Car States/5(X) -> Position_X/1
  Transformation from Raw States to Car States/6(Y) -> Position_Y/1
  Transformation from Raw States to Car States/8(Yaw_angle) -> Yaw Angle/1
  Transformation from Raw States to Car States/1(Ax) -> Acceleration_X/1
  Demux/1 -> Transformation from Raw States to Car States/1(Ax_Raw)  "Ax"
  Transformation from Raw States to Car States/4(Vy) -> Velocity_Y/1
  Demux/3 -> Transformation from Raw States to Car States/3(ddPsi)  "ddPsi"
  Demux/2 -> Transformation from Raw States to Car States/2(Ay_Raw)  "Ay"
  Gain/1 -> Dual Track Equation of Motion/1(Fx_FL)
  Gain1/1 -> Dual Track Equation of Motion/2(Fx_FR)
  Gain2/1 -> Dual Track Equation of Motion/3(Fx_RL)
  Gain3/1 -> Dual Track Equation of Motion/4(Fx_RR)
  Transformation from Raw States to Car States/2(Ay) -> Acceleration_Y/1
  Wheel_Angle/1 -> Dual Track Equation of Motion/15(Delta)
  Transformation from Raw States to Car States/9(Yaw_Rate) -> Yaw Rate/1
  Roll and Pitch/1 -> Transformation from Raw States to Car States/5(Angles)
  Az/1 -> Transformation from Raw States to Car States/4(Az)

== system egnition_New_updated_shiva/Driver Model/lateral Controller/Subsystem ==
  ey : Inport
  e_gamma : Inport  Port=2
  kappa : Inport  Port=3
  psi_dot : Inport  Port=4
  dx_C_dt : Inport  Port=5
  psi : Inport  Port=6
  Degrees to Radians : simulink_extras/Transformations/Degrees to Radians
  Gain : Constant  Value=Constants.cont_param.k_yaw
  Product : Product  Inputs=**
  Product1 : Product
  Radians to Degrees : simulink_extras/Transformations/Radians to Degrees
  Saturation : Saturate  UpperLimit=30  LowerLimit=-30
  Saturation1 : Saturate  Commented=on  UpperLimit=30  LowerLimit=-30
  Scope : Scope  Commented=on
  Stanley Gain max : Constant  Value=Constants.cont_param.k_stan
  Sum : Sum  Inputs=|++
  Trigonometric Function : Trigonometry  Operator=atan2
  dynamic Stanely : Subsystem  Commented=on
  delta_fb : Outport  VectorParamsAs1DForOutWhenUnconnected=off
  wires:
  Trigonometric Function/1 -> Sum/2
  dx_C_dt/1 -> Trigonometric Function/2, dynamic Stanely/2(v)
  Product1/1 -> Sum/1
  ey/1 -> Product/1, dynamic Stanely/1(ey)
  Product/1 -> Trigonometric Function/1
  Gain/1 -> Product1/1
  Sum/1 -> Radians to Degrees/1
  e_gamma/1 -> Product1/2
  Radians to Degrees/1 -> Saturation/1
  kappa/1 -> dynamic Stanely/3(r_meas)
  psi_dot/1 -> dynamic Stanely/4(r_trj)
  psi/1 -> dynamic Stanely/5(Yaw_c)
  dynamic Stanely/1(dynamic_steer) -> Saturation1/1  "delta"
  Stanley Gain max/1 -> Product/2
  Degrees to Radians/1 -> delta_fb/1
  Saturation1/1 -> Scope/1  "steer_dynemic"
  Saturation/1 -> Degrees to Radians/1  "steer_kinematic"

== system egnition_New_updated_shiva/Tire Forces /Tire Model/ Longitudinal  Force ==
  Fws : Inport
  Steering Angle : Inport  Port=2
  "Fwl " : Inport  Port=3
  Slip Angle : Inport  Port=4
  Bus Creator : BusCreator  Inputs=4
  Bus Selector : BusSelector  OutputSignals=Slip Angle FL,Slip Angle FR,Slip Angle RL,Slip Angle RR
  Bus Selector1 : BusSelector  OutputSignals=Fwl_FL,Fwl_FR,Fwl_RL,Fwl_RR
  Bus Selector2 : BusSelector  OutputSignals=Fws_FL,Fws_FR,Fws_RL,Fws_RR
  Demux : Demux
  MATLAB Function : MATLAB Function  TreatAsAtomicUnit=on
  Fx : Outport  VectorParamsAs1DForOutWhenUnconnected=off
  wires:
  Fws/1 -> Bus Selector2/1
  "Fwl "/1 -> Bus Selector1/1
  Slip Angle/1 -> Bus Selector/1
  Bus Selector/1 -> MATLAB Function/10(SA_FL)  "<Slip Angle FL>"
  Bus Selector/2 -> MATLAB Function/11(SA_FR)  "<Slip Angle FR>"
  Bus Selector/3 -> MATLAB Function/12(SA_RL)  "<Slip Angle RL>"
  Bus Selector/4 -> MATLAB Function/13(SA_RR)  "<Slip Angle RR>"
  Bus Selector1/1 -> MATLAB Function/6(Fwl_FL)  "<Fwl_FL>"
  Bus Selector1/2 -> MATLAB Function/7(Fwl_FR)  "<Fwl_FR>"
  Bus Selector1/3 -> MATLAB Function/8(Fwl_RL)  "<Fwl_RL>"
  Bus Selector1/4 -> MATLAB Function/9(Fwl_RR)  "<Fwl_RR>"
  Bus Selector2/1 -> MATLAB Function/2(Fws_FL)  "<Fws_FL>"
  Bus Selector2/2 -> MATLAB Function/3(Fws_FR)  "<Fws_FR>"
  Bus Selector2/3 -> MATLAB Function/4(Fws_RL)  "<Fws_RL>"
  Bus Selector2/4 -> MATLAB Function/5(Fws_RR)  "<Fws_RR>"
  Steering Angle/1 -> MATLAB Function/1(Steering_Angle)
  MATLAB Function/1(y) -> Demux/1
  Demux/4 -> Bus Creator/4  "Fx_RR"
  Demux/3 -> Bus Creator/3  "Fx_RL"
  Demux/2 -> Bus Creator/2  "Fx_FR"
  Demux/1 -> Bus Creator/1  "Fx_FL"
  Bus Creator/1 -> Fx/1

== system egnition_New_updated_shiva/Tire Forces /Tire Model/Lateral Forces ==
  Steering Angle : Inport
  Slip Angle : Inport  Port=2
  Mew : Inport  Port=3
  FZ : Inport  Port=4
  Bus Creator : BusCreator  Inputs=4
  Bus Creator1 : BusCreator  Inputs=4
  Bus Creator2 : BusCreator  Inputs=4
  Bus Selector : BusSelector  OutputSignals=Slip Angle FL,Slip Angle FR,Slip Angle RL,Slip Angle RR
  Bus Selector1 : BusSelector  OutputSignals=Mew(l)_FL,Mew(l)_FR,Mew(l)_RL,Mew(l)_RR
  Bus Selector2 : BusSelector  OutputSignals=Mew(s)_FL,Mew(s)_FR,Mew(s)_RL,Mew(s)_RR
  Bus Selector3 : BusSelector  OutputSignals=Fz_total.FZ_FL,Fz_total.FZ_FR,Fz_total.FZ_RL,Fz_total.FZ_RR
  Bus Selector4 : BusSelector  OutputSignals=Mew(l),Mew(s)
  Demux : Demux  Outputs=12
  MATLAB Function : MATLAB Function  TreatAsAtomicUnit=on
  Fy : Outport  VectorParamsAs1DForOutWhenUnconnected=off
  Fws : Outport  Port=2  VectorParamsAs1DForOutWhenUnconnected=off
  Fwl : Outport  Port=3  VectorParamsAs1DForOutWhenUnconnected=off
  wires:
  Bus Creator1/1 -> Fws/1
  Demux/5 -> Bus Creator1/1  "Fws_FL"
  Demux/6 -> Bus Creator1/2  "Fws_FR"
  Demux/7 -> Bus Creator1/3  "Fws_RL"
  Demux/8 -> Bus Creator1/4  "Fws_RR"
  Bus Creator/1 -> Fy/1
  Demux/4 -> Bus Creator/4  "Fy_RR"
  Demux/3 -> Bus Creator/3  "Fy_RL"
  Demux/2 -> Bus Creator/2  "Fy_FR"
  Demux/1 -> Bus Creator/1  "Fy_FL"
  MATLAB Function/1(y) -> Demux/1
  Bus Selector3/1 -> MATLAB Function/13(FZ_FL)  "<FZ_FL>"
  Bus Selector3/3 -> MATLAB Function/15(FZ_RL)  "<FZ_RL>"
  Bus Selector3/2 -> MATLAB Function/14(FZ_FR)  "<FZ_FR>"
  Bus Selector3/4 -> MATLAB Function/16(FZ_RR)  "<FZ_RR>"
  Bus Selector2/4 -> MATLAB Function/12(MewS_RR)  "<Mew(s)_RR>"
  Bus Selector2/3 -> MATLAB Function/11(MewS_RL)  "<Mew(s)_RL>"
  Bus Selector2/1 -> MATLAB Function/9(MewS_FL)  "<Mew(s)_FL>"
  Bus Selector2/2 -> MATLAB Function/10(MewS_FR)  "<Mew(s)_FR>"
  Bus Selector1/2 -> MATLAB Function/6(MewL_FR)  "<Mew(l)_FR>"
  Bus Selector1/3 -> MATLAB Function/7(MewL_RL)  "<Mew(l)_RL>"
  Bus Selector1/4 -> MATLAB Function/8(MewL_RR)  "<Mew(l)_RR>"
  Bus Selector1/1 -> MATLAB Function/5(MewL_FL)  "<Mew(l)_FL>"
  Bus Selector/1 -> MATLAB Function/1(SA_FL)  "<Slip Angle FL>"
  Bus Selector/2 -> MATLAB Function/2(SA_FR)  "<Slip Angle FR>"
  Bus Selector/3 -> MATLAB Function/3(SA_RL)  "<Slip Angle RL>"
  Bus Selector/4 -> MATLAB Function/4(SA_RR)  "<Slip Angle RR>"
  FZ/1 -> Bus Selector3/1
  Slip Angle/1 -> Bus Selector/1
  Steering Angle/1 -> MATLAB Function/17(Steering_Angle)
  Mew/1 -> Bus Selector4/1
  Bus Selector4/1 -> Bus Selector1/1  "<Mew(l)>"
  Bus Selector4/2 -> Bus Selector2/1  "<Mew(s)>"
  Demux/12 -> Bus Creator2/4  "Fwl_RR"
  Demux/11 -> Bus Creator2/3  "Fwl_RL"
  Demux/10 -> Bus Creator2/2  "Fwl_FR"
  Demux/9 -> Bus Creator2/1  "Fwl_FL"
  Bus Creator2/1 -> Fwl/1

== system egnition_New_updated_shiva/Tire Forces /Tire Model/Side Slip angle calculation ==
  Input Bus : Inport
  Bus Selector : BusSelector  OutputSignals=Velocity.Vx,Velocity.Vy
  Divide : Product  Inputs=/*
  Gain : Gain
  Trigonometric Function : Trigonometry  Operator=atan
  non zero : Saturate  UpperLimit=300  LowerLimit=0.00001
  Side Slip Angle : Outport  VectorParamsAs1DForOutWhenUnconnected=off
  wires:
  Divide/1 -> Trigonometric Function/1
  non zero/1 -> Divide/1
  Input Bus/1 -> Bus Selector/1
  Trigonometric Function/1 -> Gain/1
  Bus Selector/1 -> non zero/1  "<Vx>"
  Bus Selector/2 -> Divide/2  "<Vy>"
  Gain/1 -> Side Slip Angle/1

== system egnition_New_updated_shiva/Tire Forces /Tire Model/Slip angle calculation ==
  "Driver " : Inport
  Geometry_car : Inport  Port=2
  Input Bus : Inport  Port=3
  Side slip angle : Inport  Port=4
  Bus Creator : BusCreator  Inputs=4
  Bus Selector : BusSelector  OutputSignals=Velocity.Vx,Velocity.Psi_Dot
  Bus Selector1 : BusSelector  OutputSignals=Lf,Lr,Tf,Tr
  Bus Selector2 : BusSelector  OutputSignals=WheelAngle
  Demux : Demux
  MATLAB Function : MATLAB Function  TreatAsAtomicUnit=on
  Slip Angle : Outport  VectorParamsAs1DForOutWhenUnconnected=off
  wires:
  "Driver "/1 -> Bus Selector2/1
  Geometry_car/1 -> Bus Selector1/1
  Demux/4 -> Bus Creator/4  "Slip Angle RR"
  Demux/3 -> Bus Creator/3  "Slip Angle RL"
  Demux/2 -> Bus Creator/2  "Slip Angle FR"
  Demux/1 -> Bus Creator/1  "Slip Angle FL"
  Bus Creator/1 -> Slip Angle/1
  MATLAB Function/1(y) -> Demux/1
  Input Bus/1 -> Bus Selector/1
  Bus Selector/2 -> MATLAB Function/3(Yaw_Rate)  "<Psi_Dot>"
  Bus Selector/1 -> MATLAB Function/1(Velocity_COG)  "<Vx>"
  Bus Selector2/1 -> MATLAB Function/2(Steering_Angle)  "<WheelAngle>"
  Side slip angle/1 -> MATLAB Function/4(Beta)
  Bus Selector1/1 -> MATLAB Function/5(lf)  "<Lf>"
  Bus Selector1/2 -> MATLAB Function/6(lr)  "<Lr>"
  Bus Selector1/3 -> MATLAB Function/7(Tf)  "<Tf>"
  Bus Selector1/4 -> MATLAB Function/8(Tr)  "<Tr>"

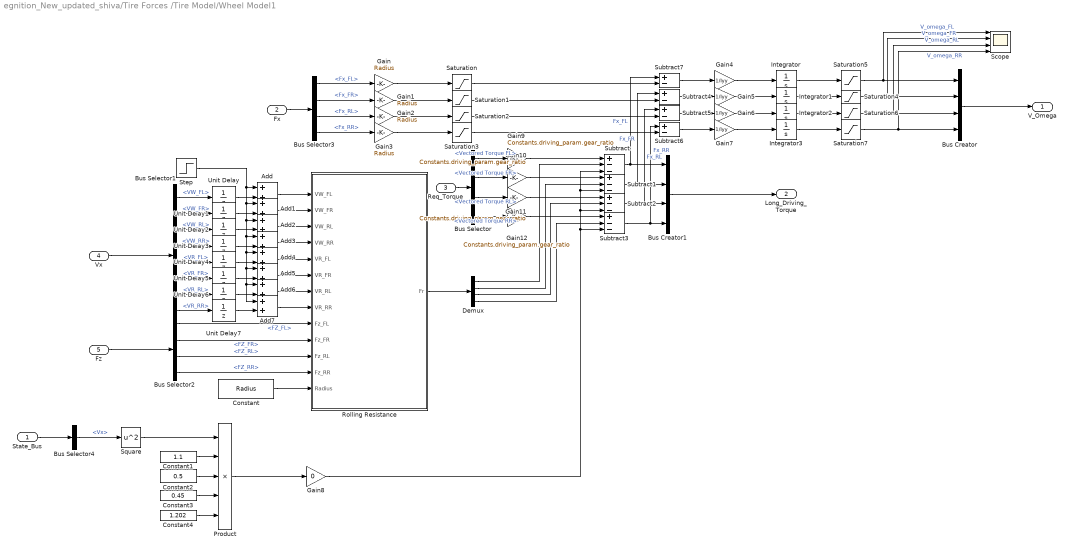
== system egnition_New_updated_shiva/Tire Forces /Tire Model/Wheel Model1 ==
  State_Bus : Inport
  Fx : Inport  Port=2
  Req_Torque : Inport  Port=3
  Vx : Inport  Port=4
  Fz : Inport  Port=5
  Add{,1..7} (8 alike) : Sum
  Bus Creator : BusCreator  Inputs=4
  Bus Creator1 : BusCreator  Inputs=4
  Bus Selector : BusSelector  OutputSignals=Vectored Torque FL,Vectored Torque FR,Vectored Torque RL,Vectored Torque RR
  Bus Selector1 : BusSelector  OutputSignals=Linear Velocity.VW_FL,Linear Velocity.VW_FR,Linear Velocity.VW_RL,Linear Velocity.VW_RR,Rotational Velocity.VR_FL,Rotational Velocity.VR_FR,Rotational Velocity.VR_RL,Rotational Velocity.VR_RR
  Bus Selector2 : BusSelector  OutputSignals=Fz_total.FZ_FL,Fz_total.FZ_FR,Fz_total.FZ_RL,Fz_total.FZ_RR
  Bus Selector3 : BusSelector  OutputSignals=Fx_FL,Fx_FR,Fx_RL,Fx_RR
  Bus Selector4 : BusSelector  OutputSignals=Velocity.Vx
  Constant : Constant  Value=Radius
  Constant1 : Constant  Value=1.1
  Constant2 : Constant  Value=0.5
  Constant3 : Constant  Value=0.45
  Constant4 : Constant  Value=1.202
  Demux : Demux
  Gain{,1..3} (4 alike) : Gain  Gain=Radius
  Gain{9..12} (4 alike) : Gain  Gain=Constants.driving_param.gear_ratio
  Gain{4..7} (4 alike) : Gain  Gain=1/Iyy
  Gain8 : Gain  Gain=0
  Integrator{,1..3} (4 alike) : Integrator
  Product : Product  Inputs=5
  Rolling Resistance : MATLAB Function  TreatAsAtomicUnit=on
  Saturation{,1..3} (4 alike) : Saturate  UpperLimit=500  LowerLimit=-500
  Saturation{4..7} (4 alike) : Saturate  UpperLimit=300  LowerLimit=-1
  Scope : Scope  NumInputPorts=4
  Square : Math  Operator=square  SaturateOnIntegerOverflow=on
  Step : Step  Time=2  Before=1  After=0
  Subtract{,1..3} (4 alike) : Sum  Inputs=+--
  Subtract{4..7} (4 alike) : Sum  Inputs=+-
  Unit Delay{,1..7} (8 alike) : UnitDelay  InitialCondition=1  SampleTime=-1  HasFrameUpgradeWarning=on
  V_Omega : Outport  VectorParamsAs1DForOutWhenUnconnected=off
  Long_Driving_Torque : Outport  Port=2  VectorParamsAs1DForOutWhenUnconnected=off
  wires:
  Gain8/1 -> Subtract2/3, Subtract/3, Subtract1/3, Subtract3/3
  Product/1 -> Gain8/1
  Square/1 -> Product/1
  Constant4/1 -> Product/5
  Constant3/1 -> Product/4
  Constant2/1 -> Product/3
  Constant1/1 -> Product/2
  Bus Selector4/1 -> Square/1  "<Vx>"
  State_Bus/1 -> Bus Selector4/1
  Rolling Resistance/1(Fr) -> Demux/1
  Bus Selector2/4 -> Rolling Resistance/12(Fz_RR)  "<FZ_RR>"
  Bus Selector2/3 -> Rolling Resistance/11(Fz_RL)  "<FZ_RL>"
  Bus Selector2/2 -> Rolling Resistance/10(Fz_FR)  "<FZ_FR>"
  Bus Selector2/1 -> Rolling Resistance/9(Fz_FL)  "<FZ_FL>"
  Fz/1 -> Bus Selector2/1
  Constant/1 -> Rolling Resistance/13(Radius)
  Subtract3/1 -> Bus Creator1/4, Subtract6/1  "Fx_RR"
  Subtract2/1 -> Bus Creator1/3, Subtract5/1  "Fx_RL"
  Subtract1/1 -> Bus Creator1/2, Subtract4/1  "Fx_FR"
  Demux/4 -> Subtract3/2
  Demux/3 -> Subtract2/2
  Demux/2 -> Subtract1/2
  Demux/1 -> Subtract/2
  Bus Selector/4 -> Gain12/1  "<Vectored Torque RR>"
  Bus Selector/3 -> Gain11/1  "<Vectored Torque RL>"
  Bus Selector/2 -> Gain10/1  "<Vectored Torque FR>"
  Bus Selector/1 -> Gain9/1  "<Vectored Torque FL>"
  Saturation3/1 -> Subtract6/2
  Saturation2/1 -> Subtract5/2
  Saturation1/1 -> Subtract4/2
  Saturation/1 -> Subtract7/2
  Saturation7/1 -> Scope/4, Bus Creator/4  "V_omega_RR"
  Saturation6/1 -> Scope/3, Bus Creator/3  "V_omega_RL"
  Saturation4/1 -> Scope/2, Bus Creator/2  "V_omega_FR"
  Saturation5/1 -> Scope/1, Bus Creator/1  "V_omega_FL"
  Gain3/1 -> Saturation3/1
  Gain2/1 -> Saturation2/1
  Gain1/1 -> Saturation1/1
  Gain/1 -> Saturation/1
  Step/1 -> Add6/1, Add7/1, Add5/1, Add4/1, Add3/1, Add2/1, Add1/1, Add/1
  Unit Delay7/1 -> Add7/2
  Unit Delay6/1 -> Add6/2
  Unit Delay5/1 -> Add5/2
  Unit Delay4/1 -> Add4/2
  Unit Delay3/1 -> Add3/2
  Unit Delay2/1 -> Add2/2
  Unit Delay1/1 -> Add1/2
  Unit Delay/1 -> Add/2
  Add7/1 -> Rolling Resistance/8(VR_RR)
  Add6/1 -> Rolling Resistance/7(VR_RL)
  Add5/1 -> Rolling Resistance/6(VR_FR)
  Add4/1 -> Rolling Resistance/5(VR_FL)
  Add3/1 -> Rolling Resistance/4(VW_RR)
  Add2/1 -> Rolling Resistance/3(VW_RL)
  Add1/1 -> Rolling Resistance/2(VW_FR)
  Add/1 -> Rolling Resistance/1(VW_FL)
  Vx/1 -> Bus Selector1/1
  Bus Selector1/8 -> Unit Delay7/1  "<VR_RR>"
  Bus Selector1/7 -> Unit Delay6/1  "<VR_RL>"
  Bus Selector1/6 -> Unit Delay5/1  "<VR_FR>"
  Bus Selector1/5 -> Unit Delay4/1  "<VR_FL>"
  Gain4/1 -> Integrator/1
  Bus Creator1/1 -> Long_Driving_Torque/1
  Subtract/1 -> Subtract7/1, Bus Creator1/1  "Fx_FL"
  Bus Creator/1 -> V_Omega/1
  Integrator/1 -> Saturation5/1
  Integrator1/1 -> Saturation4/1
  Integrator2/1 -> Saturation6/1
  Integrator3/1 -> Saturation7/1
  Subtract4/1 -> Gain5/1
  Subtract5/1 -> Gain6/1
  Subtract6/1 -> Gain7/1
  Subtract7/1 -> Gain4/1
  Bus Selector3/2 -> Gain1/1  "<Fx_FR>"
  Bus Selector3/3 -> Gain2/1  "<Fx_RL>"
  Bus Selector3/4 -> Gain3/1  "<Fx_RR>"
  Bus Selector3/1 -> Gain/1  "<Fx_FL>"
  Fx/1 -> Bus Selector3/1
  Bus Selector1/4 -> Unit Delay3/1  "<VW_RR>"
  Bus Selector1/3 -> Unit Delay2/1  "<VW_RL>"
  Bus Selector1/2 -> Unit Delay1/1  "<VW_FR>"
  Bus Selector1/1 -> Unit Delay/1  "<VW_FL>"
  Req_Torque/1 -> Bus Selector/1
  Gain5/1 -> Integrator1/1
  Gain6/1 -> Integrator2/1
  Gain7/1 -> Integrator3/1
  Gain10/1 -> Subtract1/1
  Gain9/1 -> Subtract/1
  Gain11/1 -> Subtract2/1
  Gain12/1 -> Subtract3/1

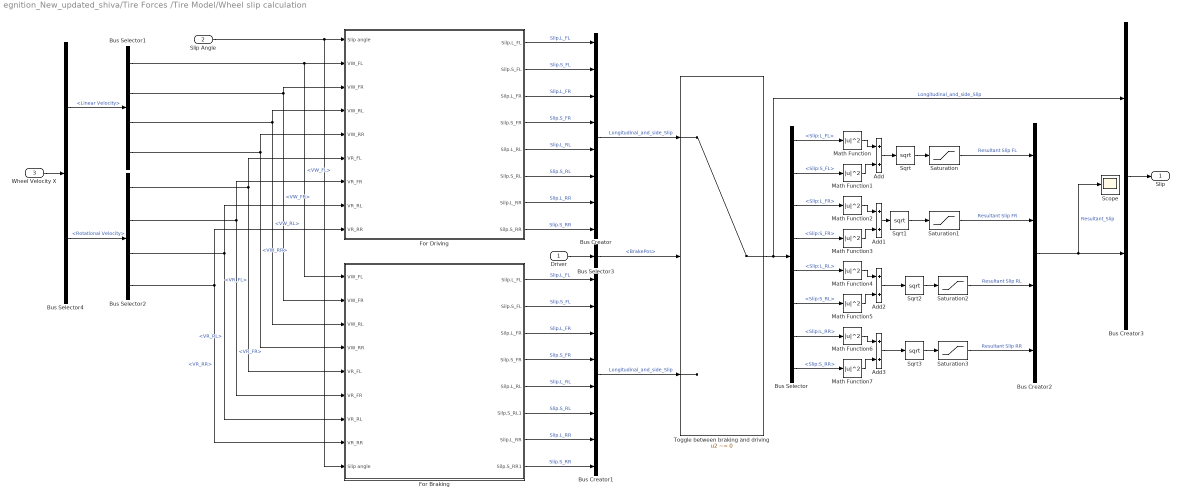
== system egnition_New_updated_shiva/Tire Forces /Tire Model/Wheel slip calculation  ==
  Driver : Inport
  "Slip Angle " : Inport  Port=2
  Wheel Velocity X : Inport  Port=3
  Add{,1..3} (4 alike) : Sum
  Bus Creator : BusCreator  Inputs=8
  Bus Creator1 : BusCreator  Inputs=8
  Bus Creator2 : BusCreator  Inputs=4
  Bus Creator3 : BusCreator  Inputs=2
  Bus Selector : BusSelector  OutputSignals=Slip:L_FL,Slip:S_FL,Slip:L_FR,Slip:S_FR,Slip:L_RL,Slip:S_RL,Slip:L_RR,Slip:S_RR
  Bus Selector1 : BusSelector  OutputSignals=VW_FL,VW_FR,VW_RL,VW_RR
  Bus Selector2 : BusSelector  OutputSignals=VR_FL,VR_FR,VR_RL,VR_RR
  Bus Selector3 : BusSelector  OutputSignals=BrakePos
  Bus Selector4 : BusSelector  OutputSignals=Linear Velocity,Rotational Velocity
  For Braking : Subsystem
  For Driving : Subsystem
  Math Function{,1..7} (8 alike) : Math  Operator=magnitude^2  SaturateOnIntegerOverflow=on
  Saturation{,1..3} (4 alike) : Saturate  UpperLimit=1  LowerLimit=0
  Scope : Scope
  Sqrt{,1..3} (4 alike) : Sqrt  SaturateOnIntegerOverflow=on
  Toggle between braking and driving : Switch  Criteria=u2 ~= 0
  " Slip" : Outport  VectorParamsAs1DForOutWhenUnconnected=off
  wires:
  Bus Creator2/1 -> Scope/1, Bus Creator3/2  "Resultant_Slip"
  Saturation3/1 -> Bus Creator2/4  "Resultant Slip RR"
  Saturation2/1 -> Bus Creator2/3  "Resultant Slip RL"
  Saturation1/1 -> Bus Creator2/2  "Resultant Slip FR"
  Saturation/1 -> Bus Creator2/1  "Resultant Slip FL"
  Bus Selector3/1 -> Toggle between braking and driving/2  "<BrakePos>"
  Driver/1 -> Bus Selector3/1
  Bus Selector4/2 -> Bus Selector2/1  "<Rotational Velocity>"
  Bus Selector1/1 -> For Driving/2("VW_FL "), For Braking/1("VW_FL ")  "<VW_FL>"
  Wheel Velocity X/1 -> Bus Selector4/1
  "Slip Angle "/1 -> For Driving/1("Slip angle "), For Braking/9("Slip angle ")
  Math Function7/1 -> Add3/2
  Sqrt3/1 -> Saturation3/1
  Add3/1 -> Sqrt3/1
  Math Function6/1 -> Add3/1
  Math Function5/1 -> Add2/2
  Sqrt2/1 -> Saturation2/1
  Add2/1 -> Sqrt2/1
  Math Function4/1 -> Add2/1
  Math Function3/1 -> Add1/2
  Sqrt1/1 -> Saturation1/1
  Add1/1 -> Sqrt1/1
  Math Function2/1 -> Add1/1
  Sqrt/1 -> Saturation/1
  Add/1 -> Sqrt/1
  Math Function1/1 -> Add/2
  Math Function/1 -> Add/1
  Bus Selector/8 -> Math Function7/1  "<Slip:S_RR>"
  Bus Selector/7 -> Math Function6/1  "<Slip:L_RR>"
  Bus Selector/6 -> Math Function5/1  "<Slip:S_RL>"
  Bus Selector/5 -> Math Function4/1  "<Slip:L_RL>"
  Bus Selector/4 -> Math Function3/1  "<Slip:S_FR>"
  Bus Selector/3 -> Math Function2/1  "<Slip:L_FR>"
  Bus Selector/2 -> Math Function1/1  "<Slip:S_FL>"
  Bus Selector/1 -> Math Function/1  "<Slip:L_FL>"
  Toggle between braking and driving/1 -> Bus Creator3/1, Bus Selector/1  "Longitudinal_and_side_Slip"
  Bus Creator1/1 -> Toggle between braking and driving/3  "Longitudinal_and_side_Slip"
  Bus Creator/1 -> Toggle between braking and driving/1  "Longitudinal_and_side_Slip"
  For Braking/5(Silp.L_RL) -> Bus Creator1/5  "Slip.L_RL"
  For Braking/6(Silp.S_RL1) -> Bus Creator1/6  "Slip.S_RL"
  For Braking/8(Silp.S_RR1) -> Bus Creator1/8  "Slip.S_RR"
  For Braking/3(Silp.L_FR) -> Bus Creator1/3  "Slip.L_FR"
  For Braking/4(Silp.S_FR) -> Bus Creator1/4  "Slip.S_FR"
  For Braking/2(Silp.S_FL) -> Bus Creator1/2  "Slip.S_FL"
  For Braking/1(Silp.L_FL) -> Bus Creator1/1  "Slip.L_FL"
  For Braking/7(Silp.L_RR) -> Bus Creator1/7  "Slip.L_RR"
  For Driving/8(Silp.S_RR) -> Bus Creator/8  "Slip.S_RR"
  For Driving/7(Silp.L_RR) -> Bus Creator/7  "Slip.L_RR"
  For Driving/6(Silp.S_RL) -> Bus Creator/6  "Slip.S_RL"
  For Driving/5(Silp.L_RL) -> Bus Creator/5  "Slip.L_RL"
  For Driving/4(Silp.S_FR) -> Bus Creator/4  "Slip.S_FR"
  For Driving/3(Silp.L_FR) -> Bus Creator/3  "Slip.L_FR"
  For Driving/2(Silp.S_FL) -> Bus Creator/2  "Slip.S_FL"
  For Driving/1(Silp.L_FL) -> Bus Creator/1  "Slip.L_FL"
  Bus Selector2/4 -> For Driving/9("VR_RR "), For Braking/8("VR_RR ")  "<VR_RR>"
  Bus Selector2/3 -> For Driving/8(VR_RL), For Braking/7(VR_RL)  "<VR_RL>"
  Bus Selector2/2 -> For Driving/7(VR_FR), For Braking/6(VR_FR)  "<VR_FR>"
  Bus Selector2/1 -> For Driving/6(VR_FL), For Braking/5(VR_FL)  "<VR_FL>"
  Bus Selector1/4 -> For Driving/5(VW_RR), For Braking/4(VW_RR)  "<VW_RR>"
  Bus Selector1/3 -> For Driving/4(VW_RL), For Braking/3(VW_RL)  "<VW_RL>"
  Bus Selector1/2 -> For Driving/3(VW_FR), For Braking/2(VW_FR)  "<VW_FR>"
  Bus Selector4/1 -> Bus Selector1/1  "<Linear Velocity>"
  Bus Creator3/1 -> " Slip"/1
